simulink model "LC_TestBench"  (R2023a)
settings: Solver=VariableStepAuto  StartTime=0.0  StopTime=10.0  RelTol=1e-3
model workspace (MAT data in the model file):
  test = Simulink.LookupTable
  test.Table = Simulink.lookuptable.Table
  test.Table.Value = [0  0.01  0.06  0.1; -0.01  0.005  0.04  0.06; -0.02  0  0.02  0.04; -0.04  0  0  0]
  test.Table.Dimensions = [4 4]
  test.Table.DataType = 'auto'
  test.Table.FieldName = 'Table'
  test.Breakpoints(1) = Simulink.lookuptable.Breakpoint
  test.Breakpoints(1).Value = [0; 40; 80; 100]
  test.Breakpoints(1).TunableSizeName = 'N1'
  test.Breakpoints(1).Dimensions = [4 1]
  test.Breakpoints(1).DataType = 'auto'
  test.Breakpoints(1).FieldName = 'BP1'
  test.Breakpoints(2) = Simulink.lookuptable.Breakpoint
  test.Breakpoints(2).Value = [0; 100; 200; 300]
  test.Breakpoints(2).TunableSizeName = 'N2'
  test.Breakpoints(2).Dimensions = [4 1]
  test.Breakpoints(2).DataType = 'auto'
  test.Breakpoints(2).FieldName = 'BP2'
  test.AllowMultipleInstancesOfTypeToHaveDifferentTableBreakpointSizes = 0
  test.SupportTunableSize = 0
  test.StructTypeInfo = Simulink.lookuptable.StructTypeInfo
  test.StructTypeInfo.Name = 'test'
  test.StructTypeInfo.DataScope = 'Auto'
settings Model: Creator=Raheel Farouk  LastModifiedBy=Raheel Farouk

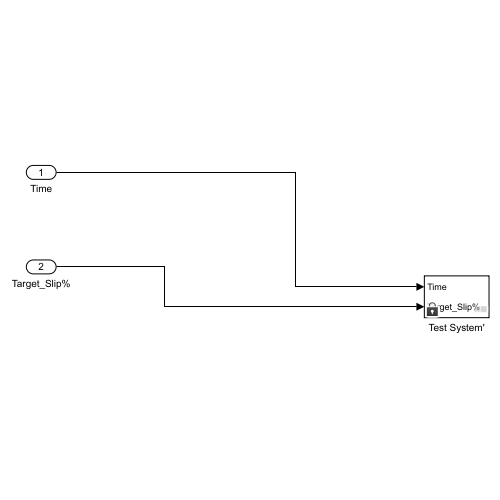
[thumbnail: Simulink's stored preview of the top-level diagram]
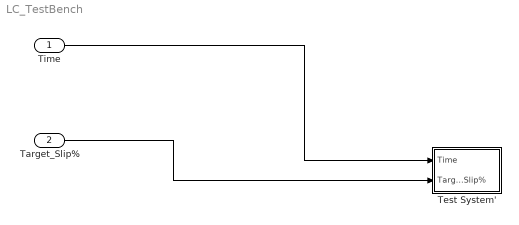
== system LC_TestBench ==
  Time : Inport
  Target_Slip% : Inport  Port=2
  Test System' : Subsystem
  wires:
  Time/1 -> Test System'/1(Time)
  Target_Slip%/1 -> Test System'/2(Target_Slip%)

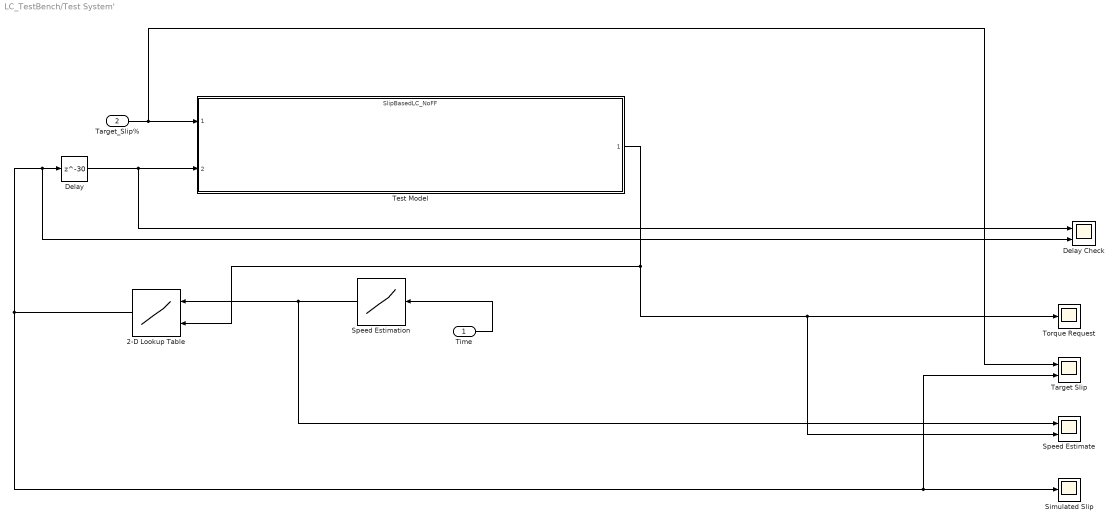
== system LC_TestBench/Test System' ==
  Time : Inport
  Target_Slip% : Inport  Port=2
  2-D Lookup Table : Lookup_n-D  DataSpecification=Lookup table object  LookupTableObject=test  BreakpointsForDimension1=[1:3]  BreakpointsForDimension2=[1:3]  InternalRulePriority=Speed  RndMeth=Simplest
      settings: InputPortMap=u0,u1
  "Delay " : Delay  DelayLength=30  InitialCondition=0
  Delay Check : Scope  NumInputPorts=2
  Simulated Slip : Scope
  Speed Estimate : Scope  NumInputPorts=2
  Speed Estimation : Lookup_n-D  NumberOfTableDimensions=1  BreakpointsForDimension1=[0;10]  Table=[0;50]  InternalRulePriority=Speed  RndMeth=Simplest
  Target Slip : Scope  NumInputPorts=2
  Test Model : ModelReference  ModelNameDialog=SlipBasedLC_NoFF.slx  SimulationMode=Normal  ModelReferenceVersion=1.31
  Torque Request : Scope
  wires:
  "Delay "/1 -> Test Model/2, Delay Check/1
  2-D Lookup Table/1 -> "Delay "/1, Delay Check/2, Simulated Slip/1, Target Slip/2
  Time/1 -> Speed Estimation/1
  Speed Estimation/1 -> 2-D Lookup Table/1, Speed Estimate/1
  Target_Slip%/1 -> Test Model/1, Target Slip/1
  Test Model/1 -> Speed Estimate/2, Torque Request/1, 2-D Lookup Table/2
